simulink model "DC_MCC"  (R2018b)
settings: Solver=FixedStepDiscrete  StartTime=0.0  StopTime=11  RelTol=1e-3  EnableMultiTasking=on
PreLoadFcn:
  | assignin('base','Ts',5e-6)
InitFcn:
  | assignin('base','Ts',5e-6)
values from neighbouring files (symbols this model uses):
  Cn = 104    [MCC.m]
  f = (phi_0*In-Cn)/Omega_n    (= 0.0113704691797)    [MCC.m]
  J = 0.12    [MCC.m]
  kc = 0    [MCC.m]
  Ki = 15    [MCC.m]
  Kw = 8    [MCC.m]
  L = 6.3e-3    (= 0.0063)    [MCC.m]
  Laf = phi_0/Ifn    (= 0.693402070952)    [MCC.m]
  Lf = 0.75*Rf    (= 102.964285714)    [MCC.m]
  Nn = 3390    [MCC.m]
  Pn = 41.4e3    (= 41400)    [MCC.m]
  R = 0.64    [MCC.m]
  Rf = Uf/Ifn    (= 137.285714286)    [MCC.m]
  to_i = L/R    (= 0.00984375)    [MCC.m]
  to_w = J/f    (= 10.5536542163)    [MCC.m]
  Uf = 310    [MCC.m]
  Un = 600    [MCC.m]
undefined symbols (not defined in the file or in its folder): DiscIntNeverNeededParam, find_system, Ts
libraries: powerlib x22, powerlib_meascontrol x3, simulink_extras x1, simulink x1
(part 1 of 2)
Description:
  | Copyright 2008-2018 The MathWorks, Inc.
settings Model: ExtModeAutoUpdateStatusClock=off  Creator=MathWorks  LastModifiedBy=Louis
settings DataIOCC: InitialState=xFinal  SaveFormat=StructureWithTime  SignalLoggingSaveFormat=ModelDataLogs  SaveOutput=off  SignalLogging=off  SaveTime=off  SignalLoggingName=sigsOut
settings OptimizationCC: BooleanDataType=off  ExpressionDepthLimit=2147483647  InitFltsAndDblsToZero=on  EfficientMapNaN2IntZero=off  LifeSpan=inf  BufferReusableBoundary=off
settings DebuggingCC: UnderspecifiedInitializationDetection=Classic  MergeDetectMultiDrivingBlocksExec=none  CheckExecutionContextPreStartOutputMsg=on  CheckExecutionContextRuntimeOutputMsg=on  SignalResolutionControl=TryResolveAllWithWarning  MultiTaskDSMMsg=warning  MultiTaskCondExecSysMsg=none  FcnCallInpInsideContextMsg=warning  BusObjectLabelMismatch=none  AllowSymbolicDim=off  StateNameClashWarn=warning  SFUnexpectedBacktrackingDiag=warning  SFNoUnconditionalDefaultTransitionDiag=warning  SFExecutionAtInitializationDiag=none
settings HardwareCC: ProdBitPerPointer=32  ProdBitPerSizeT=32  ProdBitPerPtrDiffT=32  ProdLargestAtomicFloat=None  ProdIntDivRoundTo=Undefined  ProdEndianess=Unspecified  ProdWordSize=32  ProdHWDeviceType=32-bit Generic  TargetUnknown=on
settings ModelReferenceCC: PropagateSignalLabelsOutOfModel=off
settings SFSimCC: SimUseLocalCustomCode=off
settings RTWCC: RTWUseLocalCustomCode=off
settings CodeAppCC: StateflowObjectComments=on
settings GRTTargetCC: TargetLangStandard=C89/C90 (ANSI)  GeneratePreprocessorConditionals=Disable all  CombineOutputUpdateFcns=off  GRTInterface=on
settings ConfigComp: CovMetricSettings=dw  CovHtmlReporting=on  CovSaveCumulativeToWorkspaceVar=on  CovSaveSingleToWorkspaceVar=on  CovExternalEMLEnable=off  CovSFcnEnable=off
settings SimscapeCC: SimscapeNormalizeSystem=off

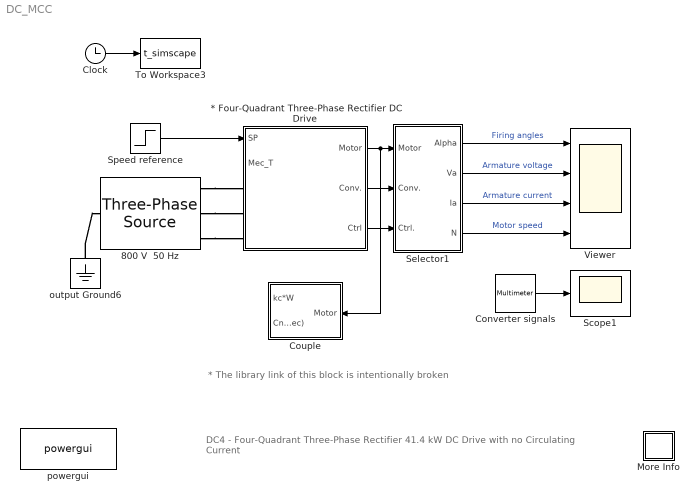
== system DC_MCC ==
  note: DC4 - Four-Quadrant Three-Phase Rectifier 41.4 kW DC Drive
      | with no Circulating Current
  note: * The library link of this block is intentionally broken
  * Four-Quadrant Three-Phase Rectifier DC Drive : Subsystem  mask(DC4){}
      mask init:
      | [X1,X1m,X2,X2m,X3,X4,Y1,Y1m,Y2,Y2m,Y3,Y4,color1,color2]=spsdrivelogo;
      mask Display:
      | patch([X1 X1m],[Y1 Y1m],color1);
      | patch(X3,Y3,color2);
      | plot([X1 X1m X2 X2m X3 X4],[Y1 Y1m Y2 Y2m Y3 Y4]);
      | text(0.5,0.3,'DC4*','HorizontalAlignment','center')
  800 V  50 Hz : powerlib/Electrical Sources/Three-Phase Source  InternalConnection=Yn  VoltagePhases=off  Voltage=800  PhaseAngle=0  Voltage_phases=[25e3 25e3 25e3]/sqrt(3)  PhaseAngles_phases=[0 -120 +120]  Frequency=50  NonIdealSource=on  SpecifyImpedance=off  Resistance=0.01  Inductance=0.1e-3  ShortCircuitLevel=0  BaseVoltage=0  XRratio=0  BusType=swing  Pref=0  Qref=0  Prefabc=0  Qrefabc=0  Qmin=-inf  Qmax=inf
      settings: SourceProductName=Simscape Electrical
  Clock : Clock
  Converter signals : powerlib/Measurements/Multimeter  PhasorSimulation=off  OutputType=Complex  sel=[10 20]  L=32  Gain=[1 1]  yselected={'Udc: * Four-Quadrant Three-Phase Rectifier DC Drive/Thyristor converter 1','Udc: * Four-Quadrant Three-Phase Rectifier DC Drive/Thyristor converter 2'};  PSBOutputType=1  PSBequivalent=0  AxesSetting=[0,0.1,-100,100]  Display=0  SavedBlockNames=-11
      settings: SourceProductName=Simscape Electrical
  Couple : Subsystem
  More Info : Subsystem
      settings: OpenFcn=showdemo(bdroot(gcb))
      mask Display: disp('?')
  Scope1 : Scope
  Selector1 : Subsystem
  Speed reference : Step  Time=4  After=Nn  SampleTime=0
  To Workspace3 : ToWorkspace  VariableName=t_simscape  SampleTime=-1
  Viewer : Scope  NumInputPorts=4
  output Ground6 : powerlib/Elements/Ground  LConnTagsString=a
      settings: SourceProductName=Simscape Electrical
  powergui : powerlib/powergui  Priority=2  SimulationMode=Discrete  SampleTime=Ts  frequency=60  Iterations=50  frequencyindice=50  Pbase=100e6  ErrMax=1e-4  UnitsV=kV  UnitsW=MW  buscounter=0  FunctionMessages=off  echomessages=off  EnableUseOfTLC=off  CurrentSourceSwitches=off  DisableSnubberDevices=off  DisableRonSwitches=off  DisableVfSwitches=off  DisplayEquations=off  SolverType=Tustin/Backward Euler (TBE)  Interpol=off  ExternalGateDelay=off  methode=off  Ts=0  x0status=blocks  SPID=off  SwTol=0  HookPort=off  RestoreLinks=warning  ResistiveCurrentMeasurement=off  Frange=[0:2:500]  Ylog=off  Xlog=on  ShowGrid=off  save=off  variable=ZData  structure=0  ZoomFFT=on  StartTime=0.0  cycles=1  DisplayStyle=1  fundamental=60  FreqAxis=off  MaxFrequency=1000  frequencyindicesteady=1  RmsSteady=1  display=off
  wires:
  Selector1/1(Alpha) -> Viewer/1  "Firing angles"
  Selector1/2(Va) -> Viewer/2  "Armature voltage"
  Selector1/3(Ia) -> Viewer/3  "Armature current"
  Selector1/4(N) -> Viewer/4  "Motor speed"
  * Four-Quadrant Three-Phase Rectifier DC Drive/1("Motor ") -> Couple/1(Motor), Selector1/1(Motor)
  * Four-Quadrant Three-Phase Rectifier DC Drive/2(Conv.) -> Selector1/2(Conv.)
  * Four-Quadrant Three-Phase Rectifier DC Drive/3(Ctrl) -> Selector1/3(Ctrl.)
  Speed reference/1 -> * Four-Quadrant Three-Phase Rectifier DC Drive/1(SP)
  Converter signals/1 -> Scope1/1
  Clock/1 -> To Workspace3/1
  connections:
  output Ground6/LConn1 -- 800 V  50 Hz/LConn1
  800 V  50 Hz/RConn1 -- * Four-Quadrant Three-Phase Rectifier DC Drive/LConn1
  800 V  50 Hz/RConn2 -- * Four-Quadrant Three-Phase Rectifier DC Drive/LConn2
  800 V  50 Hz/RConn3 -- * Four-Quadrant Three-Phase Rectifier DC Drive/LConn3

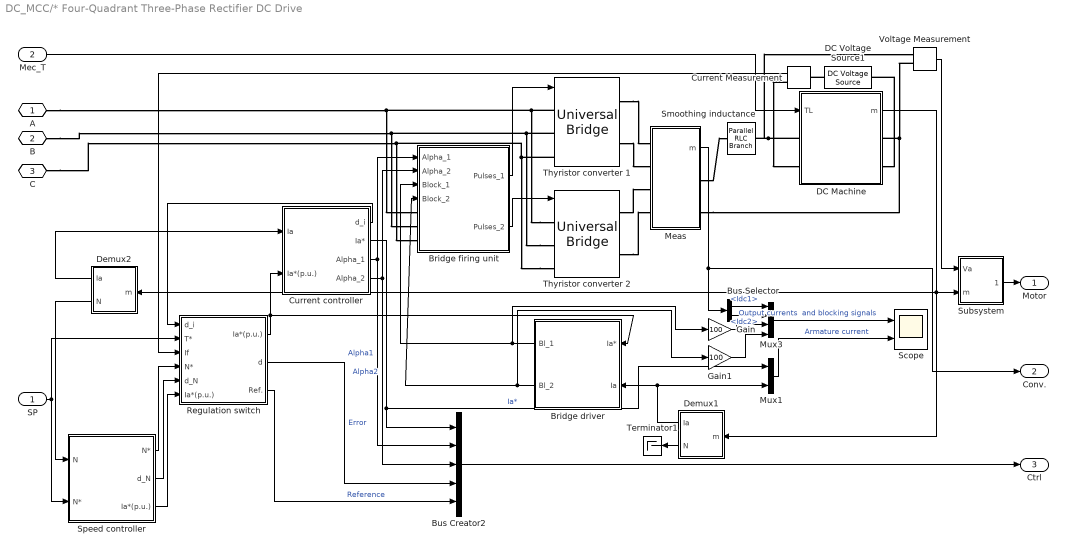
== system DC_MCC/* Four-Quadrant Three-Phase Rectifier DC Drive ==
  SP : Inport
  Mec_T : Inport  Port=2
  Bridge driver : Subsystem  mask(Bridge driver){P=Pn, V=Un, hyst=[-0.004 0.004], iazone=[0.003 0.003], irefzone=[-0.004 0.004], time=8e-3, sampling=100e-6}
      mask prompts: P "Base power (VA)"; V "Base voltage (V)"; hyst "Reference current hysteresis band [off on](p.u.)"; iazone "Armature current dead zone [low high] (p.u.)"; irefzone "Reference current dead zone [low high] (p.u.)"; time "Crossover timer delay (s)"; sampling "Controller sampling time (s)"
      mask help: This unit manages the bridge crossover process.
      mask init:
      | [X1,X1m,X2,X2m,X3,X4,Y1,Y1m,Y2,Y2m,Y3,Y4,color1,color2]=spsdrivelogo;
      | ib=P/V;
      mask Display:
      | patch([X1 X1m],[Y1 Y1m],color1);
      | patch(X3,Y3,color2);
      | plot([X1 X1m X2 X2m X3 X4],[Y1 Y1m Y2 Y2m Y3 Y4]);
  "Bridge firing unit " : Subsystem  mask(Bridge firing unit){x4=50, x9=20, Ts=Ts}
      mask prompts: x4 "Frequency of synchronisation voltages (Hz)"; x9 "Pulse width (deg.)"; Ts "Simulation time step (s)"
  Bus Creator2 : BusCreator  Inputs=5
  Bus Selector : BusSelector  OutputSignals=Idc1,Idc2
  Current Measurement : powerlib/Measurements/Current Measurement  Tag=PoWeRsYsTeMmEaSuReMeNt  PhasorSimulation=off  OutputType=Magnitude  PSBequivalent=0
      settings: SourceProductName=Simscape Electrical
  Current controller : Subsystem  Description=Current controller  mask(Current controller){Pb=Pn, Vb=Un, Kp=Ki, Ki=Ki/to_i, fci=100, lim=[20,160], sampling=100e-6, Ts=Ts}
      mask prompts: Pb "Base power (VA)"; Vb "Base voltage (V)"; Kp "Proportional gain"; Ki "Integral gain"; fci "Low-pass filter-Cut-off frequency (Hz)"; lim "Firing angle limits [ alpha_min alpha_max ] (deg.)"; sampling "Controller sampling time (s)"; Ts "Simulation time step (s)"
      mask help: This bloc implements a PI current regulator.
      mask init:
      | ib=Pb/Vb; lowlim=lim(1); highlim=lim(2);
      | [X1,X1m,X2,X2m,X3,X4,Y1,Y1m,Y2,Y2m,Y3,Y4,color1,color2]=spsdrivelogo;
      mask Display:
      | patch([X1 X1m],[Y1 Y1m],color1);
      | patch(X3,Y3,color2);
      | plot([X1 X1m X2 X2m X3 X4],[Y1 Y1m Y2 Y2m Y3 Y4]);
  DC Machine : Subsystem  LoadFcn=find_system(gcs,'FollowLinks', 'on', 'LookUnderMasks', 'all');  mask(Discrete DC machine){PresetModel=No, ShowDetailedParameters=on, RLa=[R L], RLf=[Rf Lf], Laf=Laf, J=J, Bm=f, Tf=0, w0=0, SampleTime=Ts}
      mask prompts: PresetModel "Preset  model"; ShowDetailedParameters "-----------------  Show detailed parameters -----------------"; RLa "Armature resistance and inductance [Ra (ohms) La (H) ]"; RLf "Field resistance and inductance [Rf (ohms) Lf (H) ]"; Laf "Field-armature mutual inductance Laf (H) :"; J "Total inertia J (kg.m^2)"; Bm "Viscous friction coefficient Bm (N.m.s)"; Tf "Coulomb friction torque Tf (N.m)"; w0 "Initial speed (rad/s) :"; SampleTime "Sample Time"
      mask help: This block implements a separately excited DC machine. Access is provided to the field connections so that the machine can be used as a shunt-connected or a series-connected DC machine.
      mask init:
      | Ra=RLa(1); La=RLa(2);
      | 
      | Rf=RLf(1); Lf=RLf(2);
      settings: AttributesFormatString=\n
      mask Help: helpview(psbhelp)
      mask TypeOptions PresetModel: No | 01: 5Hp 240Vdc 1750RPM Field:300Vdc | 02: 5Hp 500Vdc 1750RPM Field:300Vdc | 03: 10Hp 240Vdc 1750RPM Field:300Vdc | 04: 10Hp 500Vdc 1750RPM Field:300Vdc | 05: 20Hp 240Vdc 1750RPM Field:300Vdc | 06: 20Hp 500Vdc 1750RPM Field:300Vdc | 07: 30Hp 240Vdc 1750RPM Field:300Vdc | 08: 30Hp 500Vdc 1750RPM Field:300Vdc | 09: 40Hp 240Vdc 1750RPM Field:300Vdc | 10: 40Hp 500Vdc 1750RPM Field:300Vdc | 11: 50Hp 240Vdc 1750RPM Field:300Vdc | 12: 50Hp 500Vdc 1750RPM Field:300Vdc | 13: 75Hp 500Vdc 1750RPM Field:300Vdc | 14: 100Hp 500Vdc 1750RPM Field:300Vdc | 15: 125Hp 500Vdc 1750RPM Field:300Vdc | 16: 150Hp 500Vdc 1750RPM Field:300Vdc | 17: 175Hp 500Vdc 1750RPM Field:300Vdc | 18: 200Hp 500Vdc 1750RPM Field:300Vdc | 19: 225Hp 500Vdc 1750RPM Field:300Vdc | 20: 250Hp 500Vdc 1750RPM Field:300Vdc
      mask Callback PresetModel: powericon('DCMachineCback',gcb,'Discrete');
      mask Callback ShowDetailedParameters: powericon('DCMachineCback',gcb,'Discrete');
      mask Display:
      | plot(-80,-80,80,80,[0,9,18,24,29,30,29,24,18,9,0,-9,-18,-24,-29,-30,-29,-24,-18,-9,0],[30,29,24,18,9,0,-9,-18,-24,-29,-30,-29,-24,-18,-9,0,9,18,24,29,30],[-29,-35,-35,-29],[-8,-8,8,8],[29,35,35,29],[-8,-8,8,8],[-35,-55],[0,0],[35,55],[0,0],[-78,-50,-50,-49,-45,-39,-33,-26,-21,-18,-17,-19,-22,-22,-26,-27,-25,-22,-16,-9,-3,2,6,6,4,1,1,-3,-4,-2,2,7,14,20,26,29,30,28,24,24,21,20,21,25,31,37,44,49,50,50,50,78]*.7,[58,58,57.2,49.2,42.8,38.8,38,39.6,44.4,51.6,59.6,67.6,72.4,72.4,65.2,57.2,49.2,42.8,38.8,38,39.6,44.4,51.6,59.6,67.6,72.4,72.4,65.2,57.2,49.2,42.8,38.8,38,39.6,44.4,51.6,59.6,67.6,72.4,72.4,65.2,57.2,49.2,42.8,38.8,38,39.6,44.4,51.6,58,58,58]*.6-85 );
      | 
      | disp('dc')
      | 
      | color('blue');
      | 
      | plot([-50,-10,-10],[50,50,30]);
      | 
      | plot([50,10,10],[50,50,30]);
  DC Voltage Source1 : powerlib/Electrical Sources/DC Voltage Source  Description=source block  Amplitude=Uf  Measurements=None
      settings: AttributesFormatString=\n  SourceProductName=Simscape Electrical
  Demux1 : Subsystem
  Demux2 : Subsystem
  Gain : Gain  Gain=100  SaturateOnIntegerOverflow=on  OutDataTypeStr=Inherit: Same as input  ParamDataTypeStr=Inherit: Same as input
  Gain1 : Gain  Gain=100  SaturateOnIntegerOverflow=on  OutDataTypeStr=Inherit: Same as input  ParamDataTypeStr=Inherit: Same as input
  Meas : Subsystem
  Mux1 : Mux  Inputs=2
  Mux3 : Mux
  Regulation switch : Subsystem  mask(Regulation switch){Swk=Speed regulation, P=Pn, V=Un, Laf=Laf, lim=1, sampling=100e-6, Ts=Ts}
      mask prompts: Swk "Regulation mode"; P "Base power (VA)"; V "Base voltage (V)"; Laf "Field-armature mutual inductance Laf (H)"; lim "Current ref. limit (p.u.)"; sampling "Controller sampling time (s)"; Ts "Simulation time step (s)"
      mask help: This block allows the user to choose between speed or torque regulation.
      mask init:
      | ib=P/V;
      | [X1,X1m,X2,X2m,X3,X4,Y1,Y1m,Y2,Y2m,Y3,Y4,color1,color2]=spsdrivelogo;
      mask TypeOptions Swk: Speed regulation | Torque regulation
      mask Display:
      | patch([X1 X1m],[Y1 Y1m],color1);
      | patch(X3,Y3,color2);
      | plot([X1 X1m X2 X2m X3 X4],[Y1 Y1m Y2 Y2m Y3 Y4]);
  Scope : Scope  NumInputPorts=2
  Smoothing inductance : powerlib/Elements/Parallel RLC Branch  LConnTagsString=a  RConnTagsString=__new0  BranchType=L  Resistance=1.0  Inductance=10e-3  SetiL0=off  InitialCurrent=0  Capacitance=1.0  Setx0=off  InitialVoltage=0  Measurements=None
      settings: SourceProductName=Simscape Electrical
  Speed controller : Subsystem  mask(Speed controller){wb=Nn, ramp=[-Nn,Nn], Is=0, Kp=Kw, Ki=Kw/to_w, lim=1, fcw=40, sampling=100e-6, Ts=Ts}
      mask prompts: wb "Base speed (rpm)"; ramp "Speed reference ramp (rpm/s) [deceleration,acceleration]"; Is "Initial speed reference (rpm)"; Kp "Proportional gain"; Ki "Integral gain"; lim "Current ref. limit (p.u.)"; fcw "Low-pass filter-Cut-off frequency (Hz)"; sampling "Controller sampling time (s)"; Ts "Simulation time step (s)"
      mask help: This bloc implements a PI speed regulator.
      mask init:
      | [X1,X1m,X2,X2m,X3,X4,Y1,Y1m,Y2,Y2m,Y3,Y4,color1,color2]=spsdrivelogo;
      mask Display:
      | patch([X1 X1m],[Y1 Y1m],color1);
      | patch(X3,Y3,color2);
      | plot([X1 X1m X2 X2m X3 X4],[Y1 Y1m Y2 Y2m Y3 Y4]);
  Subsystem : Subsystem
  Terminator1 : Terminator
  Thyristor converter 1 : powerlib/Power Electronics/Universal Bridge  Arms=3  SnubberResistance=9e3  SnubberCapacitance=900e-9  Device=Thyristors  Ron=1e-3  Lon=0  ForwardVoltages="[  0,  0  ]"  ForwardVoltage=1.3  GTOparameters=[ 10e-6, 20e-6 ]  IGBTparameters=[ 1e-6 , 2e-6 ]  Measurements=All voltages and currents  Measurements_2=None  converterType=Rectifier
      settings: SourceProductName=Simscape Electrical
  Thyristor converter 2 : powerlib/Power Electronics/Universal Bridge  Arms=3  SnubberResistance=9e3  SnubberCapacitance=900e-9  Device=Thyristors  Ron=1e-3  Lon=0  ForwardVoltages="[  0,  0  ]"  ForwardVoltage=1.3  GTOparameters=[ 10e-6, 20e-6 ]  IGBTparameters=[ 1e-6 , 2e-6 ]  Measurements=All voltages and currents  Measurements_2=None  converterType=Inverter
      settings: SourceProductName=Simscape Electrical
  Voltage Measurement : powerlib/Measurements/Voltage Measurement  Tag=PoWeRsYsTeMmEaSuReMeNt  PhasorSimulation=off  OutputType=Magnitude  PSBequivalent=0
      settings: SourceProductName=Simscape Electrical
  A : PMIOPort  Side=Left
  B : PMIOPort  Port=2  Side=Left
  C : PMIOPort  Port=3  Side=Left
  "Motor " : Outport
  Conv. : Outport  Port=2
  Ctrl : Outport  Port=3
  wires:
  Current controller/4(Alpha_2) -> "Bridge firing unit "/2(Alpha_2), Bus Creator2/3  "Alpha2"
  Current controller/3(Alpha_1) -> "Bridge firing unit "/1(Alpha_1), Bus Creator2/2  "Alpha1"
  Regulation switch/3(Ref.) -> Bus Creator2/5  "Reference"
  Current controller/1(d_i) -> Regulation switch/1(d_i)
  Current controller/2(Ia*) -> Mux1/1, Bus Creator2/1  "Ia*"
  Speed controller/1(" N*") -> Regulation switch/4(N*)
  Speed controller/2(d_N) -> Regulation switch/5(d_N)
  Speed controller/3(Ia*(p.u.)) -> Regulation switch/6(Ia*(p.u.))
  Regulation switch/1(" Ia*(p.u.)") -> Current controller/2(Ia*(p.u.)), Bridge driver/1(Ia*)
  Bus Creator2/1 -> Ctrl/1
  Subsystem/1(Motor) -> "Motor "/1
  SP/1 -> Regulation switch/2(T*), Speed controller/2(N*)
  Demux2/1(Ia) -> Current controller/1(Ia)
  Demux2/2(N) -> Speed controller/1(N)
  Current Measurement/1 -> Regulation switch/3(If)
  Mec_T/1 -> DC Machine/1(TL)
  Voltage Measurement/1 -> Subsystem/1(Va)
  DC Machine/1(m) -> Demux1/1(m), Demux2/1(m), Subsystem/2(m)
  "Bridge firing unit "/1(Pulses_1) -> Thyristor converter 1/1
  "Bridge firing unit "/2(Pulses_2) -> Thyristor converter 2/1
  Demux1/1(Ia) -> Bridge driver/2(Ia), Mux1/2
  Demux1/2(N) -> Terminator1/1
  Bridge driver/1(Bl_1) -> "Bridge firing unit "/3(Block_1), Gain/1
  Bridge driver/2(Bl_2) -> "Bridge firing unit "/4(Block_2), Gain1/1
  Mux3/1 -> Scope/1  "Output currents  and blocking signals"
  Mux1/1 -> Scope/2  "Armature current"
  Gain1/1 -> Mux3/4
  Gain/1 -> Mux3/3
  Meas/1("m ") -> Conv./1, Bus Selector/1
  Bus Selector/1 -> Mux3/1  "<Idc1>"
  Bus Selector/2 -> Mux3/2  "<Idc2>"
  Regulation switch/2(d) -> Bus Creator2/4  "Error"
  connections:
  DC Machine/RConn2 -- DC Voltage Source1/LConn1
  DC Voltage Source1/RConn1 -- Current Measurement/LConn1
  Thyristor converter 2/LConn1 -- Thyristor converter 1/LConn1 -- "Bridge firing unit "/LConn1 -- A/RConn1
  Thyristor converter 2/LConn2 -- Thyristor converter 1/LConn2 -- "Bridge firing unit "/LConn2 -- B/RConn1
  Thyristor converter 2/LConn3 -- Thyristor converter 1/LConn3 -- "Bridge firing unit "/LConn3 -- C/RConn1
  Current Measurement/RConn1 -- DC Machine/LConn2
  Voltage Measurement/LConn2 -- DC Machine/RConn1 -- Meas/RConn2
  DC Machine/LConn1 -- Voltage Measurement/LConn1 -- Smoothing inductance/RConn1
  Meas/RConn1 -- Smoothing inductance/LConn1
  Thyristor converter 1/RConn1 -- Meas/LConn1
  Thyristor converter 1/RConn2 -- Meas/LConn2
  Thyristor converter 2/RConn1 -- Meas/LConn3
  Thyristor converter 2/RConn2 -- Meas/LConn4

== system DC_MCC/Couple ==
  Motor : Inport
  Demux : Demux  Outputs=5
  Gain1 : Gain  Gain=2*pi/60
  Gain2 : Gain  Gain=kc
  Step : Step  Time=6  After=Cn  SampleTime=0
  kc*W : Outport
  Cn (6sec) : Outport  Port=2
  wires:
  Motor/1 -> Demux/1
  Demux/2 -> Gain1/1
  Gain1/1 -> Gain2/1
  Gain2/1 -> kc*W/1
  Step/1 -> Cn (6sec)/1

== system DC_MCC/More Info ==

== system DC_MCC/Selector1 ==
  Motor : Inport
  Conv. : Inport  Port=2
  Ctrl. : Inport  Port=3
  Bus Selector1 : BusSelector  OutputSignals=Ia*,Reference,Alpha1,Alpha2
  Bus Selector3 : BusSelector  OutputSignals=Armature Voltage (V),Armature current ia (A),Speed (rpm)
  Mux1 : Mux  Inputs=2
  Mux2 : Mux  Inputs=2
  Mux4 : Mux  Inputs=2
  Terminator : Terminator
  Alpha : Outport
  Va : Outport  Port=2
  Ia : Outport  Port=3
  N : Outport  Port=4
  wires:
  Mux2/1 -> Ia/1
  Mux4/1 -> N/1
  Mux1/1 -> Alpha/1
  Motor/1 -> Bus Selector3/1
  Bus Selector3/1 -> Va/1  "<Armature Voltage (V)>"
  Ctrl./1 -> Bus Selector1/1
  Bus Selector1/1 -> Mux2/2  "<Ia*>"
  Bus Selector1/2 -> Mux4/2  "<Reference>"
  Bus Selector1/3 -> Mux1/1  "<Alpha1>"
  Bus Selector1/4 -> Mux1/2  "<Alpha2>"
  Bus Selector3/2 -> Mux2/1  "<Armature current ia (A)>"
  Bus Selector3/3 -> Mux4/1  "<Speed (rpm)>"
  Conv./1 -> Terminator/1

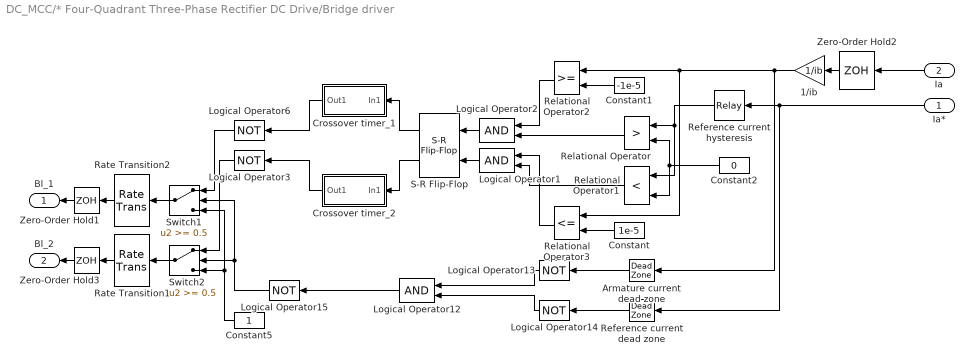
== system DC_MCC/* Four-Quadrant Three-Phase Rectifier DC Drive/Bridge driver ==
  Ia* : Inport
  Ia : Inport  Port=2
  1/ib : Gain  Gain=1/ib  SaturateOnIntegerOverflow=on  OutDataTypeStr=Inherit: Same as input  ParamDataTypeStr=Inherit: Same as input
  Armature current dead zone : DeadZone  LowerValue=iazone(1)  UpperValue=iazone(2)  SaturateOnIntegerOverflow=on
  Constant : Constant  Value=1e-5
  Constant1 : Constant  Value=-1e-5
  Constant2 : Constant  Value=0
  Constant5 : Constant
  Crossover timer_1 : Subsystem
  Crossover timer_2 : Subsystem
  Logical Operator1 : Logic
  Logical Operator12 : Logic
  Logical Operator{3,6,13..15} (5 alike) : Logic  Operator=NOT
  Logical Operator2 : Logic
  Rate Transition1 : RateTransition
  Rate Transition2 : RateTransition
  Reference current hysteresis : Relay  OnSwitchValue=hyst(2)  OffSwitchValue=hyst(1)  OffOutputValue=-1
  Reference current dead zone : DeadZone  LowerValue=irefzone(1)  UpperValue=irefzone(2)  SaturateOnIntegerOverflow=on
  Relational Operator : RelationalOperator  Operator=>  RndMeth=Nearest  InputSameDT=on
  Relational Operator1 : RelationalOperator  Operator=<  RndMeth=Nearest  InputSameDT=on
  Relational Operator2 : RelationalOperator  RndMeth=Nearest  InputSameDT=on
  Relational Operator3 : RelationalOperator  Operator=<=  RndMeth=Nearest  InputSameDT=on
  S-R Flip-Flop : simulink_extras/Flip Flops/S-R Flip-Flop  initial_condition=0
  Switch1 : Switch  Threshold=0.5  SaturateOnIntegerOverflow=on  InputSameDT=on
  Switch2 : Switch  Threshold=0.5  SaturateOnIntegerOverflow=on  InputSameDT=on
  Zero-Order Hold1 : ZeroOrderHold  SampleTime=Ts
  Zero-Order Hold2 : ZeroOrderHold  SampleTime=sampling
  Zero-Order Hold3 : ZeroOrderHold  SampleTime=Ts
  Bl_1 : Outport
  Bl_2 : Outport  Port=2
  wires:
  Relational Operator/1 -> Logical Operator2/2
  Relational Operator1/1 -> Logical Operator1/2
  Relational Operator3/1 -> Logical Operator1/1
  Relational Operator2/1 -> Logical Operator2/1
  Logical Operator6/1 -> Switch1/1
  Logical Operator3/1 -> Switch2/1
  Constant5/1 -> Switch2/3, Switch1/3
  Armature current dead zone/1 -> Logical Operator13/1
  Reference current dead zone/1 -> Logical Operator14/1
  Logical Operator13/1 -> Logical Operator12/1
  Logical Operator14/1 -> Logical Operator12/2
  Logical Operator15/1 -> Switch2/2, Switch1/2
  Logical Operator1/1 -> S-R Flip-Flop/2
  Ia*/1 -> Reference current hysteresis/1, Reference current dead zone/1
  Logical Operator12/1 -> Logical Operator15/1
  Constant1/1 -> Relational Operator2/2
  Constant/1 -> Relational Operator3/2
  Constant2/1 -> Relational Operator1/2, Relational Operator/2
  Ia/1 -> Zero-Order Hold2/1
  Logical Operator2/1 -> S-R Flip-Flop/1
  S-R Flip-Flop/2 -> Crossover timer_2/1(In1)
  S-R Flip-Flop/1 -> Crossover timer_1/1(In1)
  Zero-Order Hold1/1 -> Bl_1/1
  Crossover timer_2/1(Out1) -> Logical Operator3/1
  Zero-Order Hold3/1 -> Bl_2/1
  Switch2/1 -> Rate Transition1/1
  Rate Transition1/1 -> Zero-Order Hold3/1
  Crossover timer_1/1(Out1) -> Logical Operator6/1
  Zero-Order Hold2/1 -> 1/ib/1
  1/ib/1 -> Relational Operator3/1, Relational Operator2/1, Armature current dead zone/1
  Switch1/1 -> Rate Transition2/1
  Rate Transition2/1 -> Zero-Order Hold1/1
  Reference current hysteresis/1 -> Relational Operator/1, Relational Operator1/1

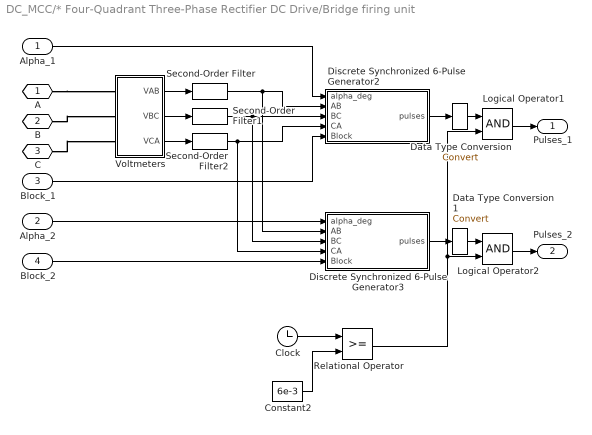
== system DC_MCC/* Four-Quadrant Three-Phase Rectifier DC Drive/Bridge firing unit  ==
  Alpha_1 : Inport
  Alpha_2 : Inport  Port=2
  Block_1 : Inport  Port=3
  Block_2 : Inport  Port=4
  Clock : Clock
  Constant2 : Constant  Value=6e-3
  Data Type Conversion : DataTypeConversion  SaturateOnIntegerOverflow=on  RndMeth=Zero
  Data Type Conversion1 : DataTypeConversion  SaturateOnIntegerOverflow=on  RndMeth=Zero
  Discrete Synchronized 6-Pulse Generator2 : Subsystem  mask(Discrete Synchronized 6-pulse generator){freq=x4, pwidth=x9, Double_Pulse=on, Ts=Ts}
      mask prompts: freq "Frequency of sync. voltages (Hz):"; pwidth "Pulse width (degrees) :"; Double_Pulse "Double pulsing"; Ts "Time step (s) :"
      mask help:
      | Use this block to fire the 6 thyristors of a 6-pulse converter.
      |
      | The output is a vector of 6 pulses (0-1) individually synchronized on the 6 commutation voltages. Pulses are generated alpha degrees after the increasing zero-crossings of the commutation voltages.
      |
      | Input 1 is  the alpha firing signal (degrees).
      | Inputs 2, 3 and 4 are the synchronization voltages AB BC CA which should be in phase with the 3 phase-phase voltages at the converter terminals.
      | Input 5: Frequency of the synchronization voltages (use a constant or the Freq PLL output)
      | Input 6 allows  blocking of the pulses when the applied signal is non zero.
      |
      | When the 'Douple pulsing' option is checked, two pulses are sent to each thyristor: a 1st pulse when the aplha angle is reached, then a 2nd pulse 60 degrees later, when the next thyristor is fired.
      mask Display: plot(0,0,100,100,[80 62 62 47 47 30],[40 40 60 60 40 40]-5)
  Discrete Synchronized 6-Pulse Generator3 : Subsystem  mask(Discrete Synchronized 6-pulse generator){freq=x4, pwidth=x9, Double_Pulse=on, Ts=Ts}
      mask prompts: freq "Frequency of sync. voltages (Hz):"; pwidth "Pulse width (degrees) :"; Double_Pulse "Double pulsing"; Ts "Time step (s) :"
      mask help:
      | Use this block to fire the 6 thyristors of a 6-pulse converter.
      |
      | The output is a vector of 6 pulses (0-1) individually synchronized on the 6 commutation voltages. Pulses are generated alpha degrees after the increasing zero-crossings of the commutation voltages.
      |
      | Input 1 is  the alpha firing signal (degrees).
      | Inputs 2, 3 and 4 are the synchronization voltages AB BC CA which should be in phase with the 3 phase-phase voltages at the converter terminals.
      | Input 5: Frequency of the synchronization voltages (use a constant or the Freq PLL output)
      | Input 6 allows  blocking of the pulses when the applied signal is non zero.
      |
      | When the 'Douple pulsing' option is checked, two pulses are sent to each thyristor: a 1st pulse when the aplha angle is reached, then a 2nd pulse 60 degrees later, when the next thyristor is fired.
      mask Display: plot(0,0,100,100,[80 62 62 47 47 30],[40 40 60 60 40 40]-5)
  Logical Operator1 : Logic
  Logical Operator2 : Logic
  Relational Operator : RelationalOperator  RndMeth=Nearest  InputSameDT=on
  Second-Order Filter : powerlib_meascontrol/Filters/Second-Order Filter  FilterType=Bandpass  Fo=x4  Zeta=0.25  Ts=Ts  Initialize=off  Vac_Init="[0,  0,  60]"  Vdc_Init=0  PlotResponse=off  FreqRange=[0, 500, 1]
      settings: SourceProductName=Simscape Electrical  SourceProductBaseCode=PS
  Second-Order Filter1 : powerlib_meascontrol/Filters/Second-Order Filter  FilterType=Bandpass  Fo=x4  Zeta=0.25  Ts=Ts  Initialize=on  Vac_Init=[0.8 -25 60]  Vdc_Init=-0.4  PlotResponse=off  FreqRange=[0, 500, 1]
      settings: SourceProductName=Simscape Electrical  SourceProductBaseCode=PS
  Second-Order Filter2 : powerlib_meascontrol/Filters/Second-Order Filter  FilterType=Bandpass  Fo=x4  Zeta=0.25  Ts=Ts  Initialize=on  Vac_Init=[0.8 -25 60]  Vdc_Init=-0.4  PlotResponse=off  FreqRange=[0, 500, 1]
      settings: SourceProductName=Simscape Electrical  SourceProductBaseCode=PS
  Voltmeters : Subsystem
  A : PMIOPort  Side=Left
  B : PMIOPort  Port=2  Side=Left
  C : PMIOPort  Port=3  Side=Left
  Pulses_1 : Outport
  Pulses_2 : Outport  Port=2
  wires:
  Discrete Synchronized 6-Pulse Generator3/1(pulses) -> Data Type Conversion1/1
  Logical Operator2/1 -> Pulses_2/1
  Discrete Synchronized 6-Pulse Generator2/1(pulses) -> Data Type Conversion/1
  Logical Operator1/1 -> Pulses_1/1
  Relational Operator/1 -> Logical Operator1/2, Logical Operator2/2
  Constant2/1 -> Relational Operator/2
  Clock/1 -> Relational Operator/1
  Voltmeters/1(VAB) -> Second-Order Filter/1
  Voltmeters/2(VBC) -> Second-Order Filter1/1
  Voltmeters/3(VCA) -> Second-Order Filter2/1
  Alpha_1/1 -> Discrete Synchronized 6-Pulse Generator2/1(alpha_deg)
  Second-Order Filter/1 -> Discrete Synchronized 6-Pulse Generator2/2(AB), Discrete Synchronized 6-Pulse Generator3/2(AB)
  Second-Order Filter1/1 -> Discrete Synchronized 6-Pulse Generator2/3(BC), Discrete Synchronized 6-Pulse Generator3/3(BC)
  Second-Order Filter2/1 -> Discrete Synchronized 6-Pulse Generator2/4(CA), Discrete Synchronized 6-Pulse Generator3/4(CA)
  Alpha_2/1 -> Discrete Synchronized 6-Pulse Generator3/1(alpha_deg)
  Block_1/1 -> Discrete Synchronized 6-Pulse Generator2/5(Block)
  Block_2/1 -> Discrete Synchronized 6-Pulse Generator3/5(Block)
  Data Type Conversion/1 -> Logical Operator1/1
  Data Type Conversion1/1 -> Logical Operator2/1
  connections:
  A/RConn1 -- Voltmeters/LConn1
  B/RConn1 -- Voltmeters/LConn2
  C/RConn1 -- Voltmeters/LConn3

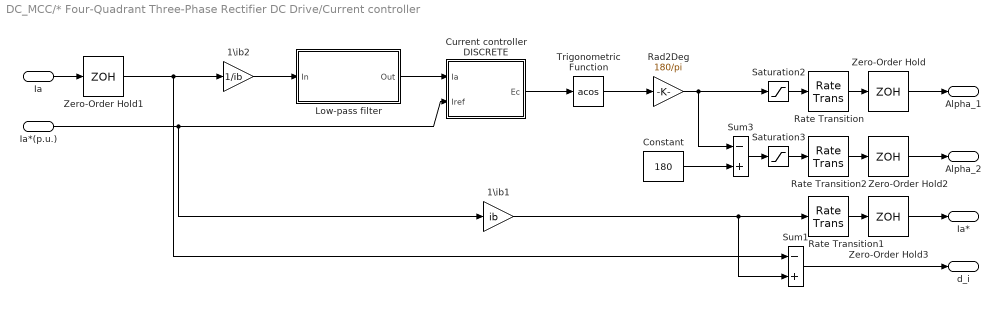
== system DC_MCC/* Four-Quadrant Three-Phase Rectifier DC Drive/Current controller ==
  Ia : Inport
  Ia*(p.u.) : Inport  Port=2
  1\ib1 : Gain  Gain=ib  SaturateOnIntegerOverflow=on  OutDataTypeStr=Inherit: Same as input  ParamDataTypeStr=Inherit: Same as input
  1\ib2 : Gain  Gain=1/ib  SaturateOnIntegerOverflow=on  OutDataTypeStr=Inherit: Same as input  ParamDataTypeStr=Inherit: Same as input
  Constant : Constant  Value=180
  Current controller DISCRETE : Subsystem  mask(PI controller){Kp=Kp, Ki=Ki, Ts=sampling}
      mask prompts: Kp "Proportional gain (Kp)"; Ki "Integral gain (Ki)"; Ts "Sample time (s) :"
      mask help: Proportional-Integral Speed Controller
      mask Display: plot(0,0,100,100,[35,35,65],[70,30,30],[35,65],[45,60])
  Low-pass filter : Subsystem
  Rad2Deg : Gain  Gain=180/pi  SaturateOnIntegerOverflow=on  OutDataTypeStr=Inherit: Same as input  ParamDataTypeStr=Inherit: Same as input
  Rate Transition : RateTransition
  Rate Transition1 : RateTransition
  Rate Transition2 : RateTransition
  Saturation2 : Saturate  UpperLimit=highlim  LowerLimit=lowlim
  Saturation3 : Saturate  UpperLimit=highlim  LowerLimit=lowlim
  Sum1 : Sum  Inputs=-+  SaturateOnIntegerOverflow=on  InputSameDT=on  OutDataTypeStr=Inherit: Same as first input
  Sum3 : Sum  Inputs=-+  SaturateOnIntegerOverflow=on  InputSameDT=on  OutDataTypeStr=Inherit: Same as first input
  Trigonometric Function : Trigonometry  Operator=acos
  Zero-Order Hold : ZeroOrderHold  SampleTime=Ts
  Zero-Order Hold1 : ZeroOrderHold  SampleTime=sampling
  Zero-Order Hold2 : ZeroOrderHold  SampleTime=Ts
  Zero-Order Hold3 : ZeroOrderHold  SampleTime=Ts
  d_i : Outport
  Ia* : Outport  Port=2
  Alpha_1 : Outport  Port=3
  Alpha_2 : Outport  Port=4
  wires:
  Rad2Deg/1 -> Saturation2/1, Sum3/1
  Trigonometric Function/1 -> Rad2Deg/1
  Current controller DISCRETE/1(Ec) -> Trigonometric Function/1
  Ia*(p.u.)/1 -> 1\ib1/1, Current controller DISCRETE/2(Iref)
  Low-pass filter/1(Out) -> Current controller DISCRETE/1(Ia)
  1\ib2/1 -> Low-pass filter/1(In)
  Zero-Order Hold1/1 -> Sum1/1, 1\ib2/1
  Ia/1 -> Zero-Order Hold1/1
  Sum1/1 -> d_i/1
  Zero-Order Hold/1 -> Alpha_1/1
  Saturation2/1 -> Rate Transition/1
  Rate Transition1/1 -> Zero-Order Hold3/1
  Zero-Order Hold3/1 -> Ia*/1
  Rate Transition/1 -> Zero-Order Hold/1
  1\ib1/1 -> Sum1/2, Rate Transition1/1
  Saturation3/1 -> Rate Transition2/1
  Zero-Order Hold2/1 -> Alpha_2/1
  Constant/1 -> Sum3/2
  Rate Transition2/1 -> Zero-Order Hold2/1
  Sum3/1 -> Saturation3/1

== system DC_MCC/* Four-Quadrant Three-Phase Rectifier DC Drive/DC Machine ==
  TL : Inport
  FCEM : powerlib/Electrical Sources/Controlled Voltage Source  Description=source block  Initialize=on  Source_Type=AC  Amplitude=0  Phase=0  Frequency=0  Measurements=None
      settings: SourceProductName=Simscape Electrical
  Measurement list : Subsystem
  Mechanics : Subsystem
  Ra La : powerlib/Elements/Series RLC Branch  LConnTagsString=__new0  RConnTagsString=__new0  BranchType=RL  Resistance=Ra  Inductance=La  SetiL0=off  InitialCurrent=0  Capacitance=1.0  Setx0=off  InitialVoltage=0  Measurements=None
      settings: SourceProductName=Simscape Electrical
  Rf  Lf : powerlib/Elements/Series RLC Branch  LConnTagsString=__new0  RConnTagsString=__new0  BranchType=RL  Resistance=Rf  Inductance=Lf  SetiL0=off  InitialCurrent=0  Capacitance=1.0  Setx0=off  InitialVoltage=0  Measurements=None
      settings: SourceProductName=Simscape Electrical
  iA : powerlib/Measurements/Current Measurement  PhasorSimulation=off  OutputType=Magnitude  PSBequivalent=0
      settings: SourceProductName=Simscape Electrical
  iF : powerlib/Measurements/Current Measurement  PhasorSimulation=off  OutputType=Magnitude  PSBequivalent=0
      settings: SourceProductName=Simscape Electrical
  A+ : PMIOPort  Side=Left
  A- : PMIOPort  Port=2  Side=Right
  F+ : PMIOPort  Port=3  Side=Left
  F- : PMIOPort  Port=4  Side=Right
  m : Outport
  wires:
  Measurement list/1(Out1) -> m/1
  Mechanics/1(m) -> Measurement list/1(In1)
  TL/1 -> Mechanics/1(TL)
  iF/1 -> Mechanics/3(iF)
  Mechanics/2(FCEM) -> FCEM/1
  iA/1 -> Mechanics/2(iA)
  connections:
  F-/RConn1 -- Rf  Lf/RConn1
  F+/RConn1 -- iF/LConn1
  A-/RConn1 -- FCEM/LConn1
  A+/RConn1 -- iA/LConn1
  iF/RConn1 -- Rf  Lf/LConn1
  iA/RConn1 -- Ra La/LConn1
  FCEM/RConn1 -- Ra La/RConn1

== system DC_MCC/* Four-Quadrant Three-Phase Rectifier DC Drive/Demux1 ==
  m : Inport
  Demux : Demux
  Rad2Rpm : Gain  Gain=30/pi  SaturateOnIntegerOverflow=on  OutDataTypeStr=Inherit: Same as input  ParamDataTypeStr=Inherit: Same as input
  Terminator : Terminator
  Terminator1 : Terminator
  Ia : Outport
  N : Outport  Port=2
  wires:
  Demux/4 -> Terminator1/1
  Demux/3 -> Terminator/1
  m/1 -> Demux/1
  Demux/2 -> Ia/1
  Demux/1 -> Rad2Rpm/1
  Rad2Rpm/1 -> N/1

== system DC_MCC/* Four-Quadrant Three-Phase Rectifier DC Drive/Demux2 ==
  m : Inport
  Demux : Demux
  Rad2Rpm : Gain  Gain=30/pi  SaturateOnIntegerOverflow=on  OutDataTypeStr=Inherit: Same as input  ParamDataTypeStr=Inherit: Same as input
  Terminator : Terminator
  Terminator1 : Terminator
  Ia : Outport
  N : Outport  Port=2
  wires:
  Demux/4 -> Terminator1/1
  Demux/3 -> Terminator/1
  m/1 -> Demux/1
  Demux/2 -> Ia/1
  Demux/1 -> Rad2Rpm/1
  Rad2Rpm/1 -> N/1

== system DC_MCC/* Four-Quadrant Three-Phase Rectifier DC Drive/Meas ==
  Bus Creator2 : BusCreator  Inputs=4
  Current Measurement3 : powerlib/Measurements/Current Measurement  Tag=PoWeRsYsTeMmEaSuReMeNt  PhasorSimulation=off  OutputType=Magnitude  PSBequivalent=0
      settings: SourceProductName=Simscape Electrical
  Current Measurement4 : powerlib/Measurements/Current Measurement  Tag=PoWeRsYsTeMmEaSuReMeNt  PhasorSimulation=off  OutputType=Magnitude  PSBequivalent=0
      settings: SourceProductName=Simscape Electrical
  Voltage Measurement1 : powerlib/Measurements/Voltage Measurement  Tag=PoWeRsYsTeMmEaSuReMeNt  PhasorSimulation=off  OutputType=Magnitude  PSBequivalent=0
      settings: SourceProductName=Simscape Electrical
  Voltage Measurement2 : powerlib/Measurements/Voltage Measurement  Tag=PoWeRsYsTeMmEaSuReMeNt  PhasorSimulation=off  OutputType=Magnitude  PSBequivalent=0
      settings: SourceProductName=Simscape Electrical
  1+ : PMIOPort  Side=Left
  1_out : PMIOPort  Port=2  Side=Right
  1- : PMIOPort  Port=3  Side=Left
  2+ : PMIOPort  Port=4  Side=Left
  2_out : PMIOPort  Port=5  Side=Right
  2- : PMIOPort  Port=6  Side=Left
  "m " : Outport
  wires:
  Voltage Measurement1/1 -> Bus Creator2/1  "Vdc1"
  Voltage Measurement2/1 -> Bus Creator2/2  "Vdc2"
  Current Measurement4/1 -> Bus Creator2/3  "Idc1"
  Current Measurement3/1 -> Bus Creator2/4  "Idc2"
  Bus Creator2/1 -> "m "/1
  connections:
  1+/RConn1 -- Current Measurement4/LConn1 -- Voltage Measurement1/LConn1
  2_out/RConn1 -- Current Measurement3/RConn1 -- Voltage Measurement1/LConn2 -- 1-/RConn1
  2+/RConn1 -- Current Measurement3/LConn1 -- Voltage Measurement2/LConn1
  Voltage Measurement2/LConn2 -- Current Measurement4/RConn1 -- 1_out/RConn1 -- 2-/RConn1

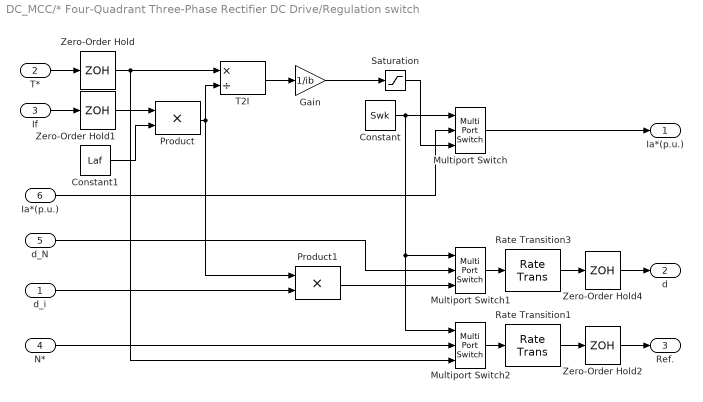
== system DC_MCC/* Four-Quadrant Three-Phase Rectifier DC Drive/Regulation switch ==
  d_i : Inport
  T* : Inport  Port=2
  If : Inport  Port=3
  N* : Inport  Port=4
  d_N : Inport  Port=5
  Ia*(p.u.) : Inport  Port=6
  Constant : Constant  Value=Swk
  Constant1 : Constant  Value=Laf
  Gain : Gain  Gain=1/ib  SaturateOnIntegerOverflow=on  OutDataTypeStr=Inherit: Same as input  ParamDataTypeStr=Inherit: Same as input
  Multiport Switch : MultiPortSwitch  Inputs=2  SaturateOnIntegerOverflow=on
  Multiport Switch1 : MultiPortSwitch  Inputs=2  SaturateOnIntegerOverflow=on
  Multiport Switch2 : MultiPortSwitch  Inputs=2  SaturateOnIntegerOverflow=on
  Product : Product  SaturateOnIntegerOverflow=on  OutDataTypeStr=Inherit: Same as first input
  Product1 : Product  SaturateOnIntegerOverflow=on  OutDataTypeStr=Inherit: Same as first input
  Rate Transition1 : RateTransition
  Rate Transition3 : RateTransition
  Saturation : Saturate  UpperLimit=lim  LowerLimit=-lim
  T2I : Product  Inputs=*/  SaturateOnIntegerOverflow=on  OutDataTypeStr=Inherit: Same as first input
  Zero-Order Hold : ZeroOrderHold  SampleTime=sampling
  Zero-Order Hold1 : ZeroOrderHold  SampleTime=sampling
  Zero-Order Hold2 : ZeroOrderHold  SampleTime=Ts
  Zero-Order Hold4 : ZeroOrderHold  SampleTime=Ts
  " Ia*(p.u.)" : Outport
  d : Outport  Port=2
  Ref. : Outport  Port=3
  wires:
  Product1/1 -> Multiport Switch1/3
  d_N/1 -> Multiport Switch1/2
  T2I/1 -> Gain/1
  Saturation/1 -> Multiport Switch/3
  Gain/1 -> Saturation/1
  Zero-Order Hold/1 -> Multiport Switch2/3, T2I/1
  T*/1 -> Zero-Order Hold/1
  If/1 -> Zero-Order Hold1/1
  Constant/1 -> Multiport Switch2/1, Multiport Switch1/1, Multiport Switch/1
  Zero-Order Hold1/1 -> Product/1
  Product/1 -> T2I/2, Product1/1
  Constant1/1 -> Product/2
  Rate Transition3/1 -> Zero-Order Hold4/1
  Zero-Order Hold4/1 -> d/1
  Multiport Switch1/1 -> Rate Transition3/1
  d_i/1 -> Product1/2
  Rate Transition1/1 -> Zero-Order Hold2/1
  Zero-Order Hold2/1 -> Ref./1
  Multiport Switch2/1 -> Rate Transition1/1
  N*/1 -> Multiport Switch2/2
  Multiport Switch/1 -> " Ia*(p.u.)"/1
  Ia*(p.u.)/1 -> Multiport Switch/2

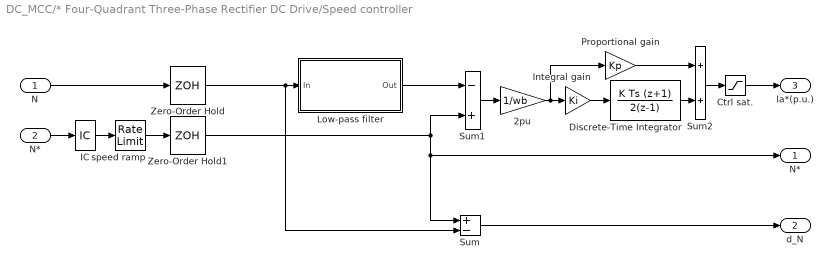
== system DC_MCC/* Four-Quadrant Three-Phase Rectifier DC Drive/Speed controller ==
  N : Inport
  N* : Inport  Port=2
  2pu : Gain  Gain=1/wb  SaturateOnIntegerOverflow=on  OutDataTypeStr=Inherit: Same as input  ParamDataTypeStr=Inherit: Same as input
  Ctrl sat. : Saturate  UpperLimit=lim  LowerLimit=-lim
  Discrete-Time Integrator : DiscreteIntegrator  IntegratorMethod=Integration: Trapezoidal  SampleTime=sampling  LimitOutput=on  UpperSaturationLimit=lim  LowerSaturationLimit=-lim  ICPrevOutput=DiscIntNeverNeededParam  ICPrevScaledInput=DiscIntNeverNeededParam
  IC : InitialCondition  Value=Is
  Integral gain : Gain  Gain=Ki  SaturateOnIntegerOverflow=on  OutDataTypeStr=Inherit: Same as input  ParamDataTypeStr=Inherit: Same as input
  Low-pass filter : Subsystem
  Proportional gain : Gain  Gain=Kp  SaturateOnIntegerOverflow=on  OutDataTypeStr=Inherit: Same as input  ParamDataTypeStr=Inherit: Same as input
  Sum : Sum  Inputs=+-  SaturateOnIntegerOverflow=on  InputSameDT=on  OutDataTypeStr=Inherit: Same as first input
  Sum1 : Sum  Inputs=-+  SaturateOnIntegerOverflow=on  InputSameDT=on  OutDataTypeStr=Inherit: Same as first input
  Sum2 : Sum  SaturateOnIntegerOverflow=on  InputSameDT=on  OutDataTypeStr=Inherit: Same as first input
  Zero-Order Hold : ZeroOrderHold  SampleTime=sampling
  Zero-Order Hold1 : ZeroOrderHold  SampleTime=sampling
  speed ramp : RateLimiter  RisingSlewLimit=ramp(2)  FallingSlewLimit=ramp(1)
  " N*" : Outport  InitialOutput=0
  d_N : Outport  Port=2  InitialOutput=0
  Ia*(p.u.) : Outport  Port=3  InitialOutput=0
  wires:
  speed ramp/1 -> Zero-Order Hold1/1
  Ctrl sat./1 -> Ia*(p.u.)/1
  2pu/1 -> Integral gain/1, Proportional gain/1
  Sum1/1 -> 2pu/1
  Proportional gain/1 -> Sum2/1
  Integral gain/1 -> Discrete-Time Integrator/1
  Discrete-Time Integrator/1 -> Sum2/2
  Sum2/1 -> Ctrl sat./1
  Sum/1 -> d_N/1
  Low-pass filter/1(Out) -> Sum1/1
  N*/1 -> IC/1
  IC/1 -> speed ramp/1
  N/1 -> Zero-Order Hold/1
  Zero-Order Hold/1 -> Sum/2, Low-pass filter/1(In)
  Zero-Order Hold1/1 -> " N*"/1, Sum/1, Sum1/2

== system DC_MCC/* Four-Quadrant Three-Phase Rectifier DC Drive/Subsystem ==
  Va : Inport
  m : Inport  Port=2
  1\ib1 : Gain  Gain=30/pi  SaturateOnIntegerOverflow=on  OutDataTypeStr=Inherit: Same as input  ParamDataTypeStr=Inherit: Same as input
  Bus Creator3 : BusCreator  Inputs=5
  Bus Selector : BusSelector  OutputSignals=Speed wm (rad/s),Armature current ia (A),Field current if (A),Electrical torque Te (n m)
  Motor : Outport
  wires:
  Bus Selector/1 -> 1\ib1/1  "<Speed wm (rad/s)>"
  m/1 -> Bus Selector/1
  Va/1 -> Bus Creator3/1  "Armature Voltage (V)"
  Bus Creator3/1 -> Motor/1
  Bus Selector/2 -> Bus Creator3/3  "<Armature current ia (A)>"
  Bus Selector/3 -> Bus Creator3/4  "<Field current if (A)>"
  1\ib1/1 -> Bus Creator3/2  "Speed (rpm)"
  Bus Selector/4 -> Bus Creator3/5  "<Electrical torque Te (n m)>"

== system DC_MCC/* Four-Quadrant Three-Phase Rectifier DC Drive/Bridge driver/Crossover timer_1 ==
  In1 : Inport
  Constant3 : Constant  Value=time
  Digital Clock : DigitalClock  SampleTime=sampling
  Logical Operator15 : Logic  Operator=NOT
  Relational Operator4 : RelationalOperator  Operator=>  RndMeth=Nearest  InputSameDT=on
  Sum2 : Sum  Inputs=+-  SaturateOnIntegerOverflow=on  InputSameDT=on  OutDataTypeStr=Inherit: Same as first input
  Switch3 : Switch  Threshold=0.5  SaturateOnIntegerOverflow=on  InputSameDT=on
  Unit Delay2 : UnitDelay  SampleTime=sampling
  Out1 : Outport
  wires:
  Logical Operator15/1 -> Switch3/2
  In1/1 -> Logical Operator15/1
  Relational Operator4/1 -> Out1/1
  Constant3/1 -> Relational Operator4/2
  Sum2/1 -> Relational Operator4/1
  Unit Delay2/1 -> Switch3/3
  Digital Clock/1 -> Sum2/1, Switch3/1
  Switch3/1 -> Sum2/2, Unit Delay2/1

== system DC_MCC/* Four-Quadrant Three-Phase Rectifier DC Drive/Bridge driver/Crossover timer_2 ==
  In1 : Inport
  Constant3 : Constant  Value=time
  Digital Clock : DigitalClock  SampleTime=sampling
  Logical Operator15 : Logic  Operator=NOT
  Relational Operator4 : RelationalOperator  Operator=>  RndMeth=Nearest  InputSameDT=on
  Sum2 : Sum  Inputs=+-  SaturateOnIntegerOverflow=on  InputSameDT=on  OutDataTypeStr=Inherit: Same as first input
  Switch3 : Switch  Threshold=0.5  SaturateOnIntegerOverflow=on  InputSameDT=on
  Unit Delay2 : UnitDelay  SampleTime=sampling
  Out1 : Outport
  wires:
  Switch3/1 -> Unit Delay2/1, Sum2/2
  Digital Clock/1 -> Switch3/1, Sum2/1
  Unit Delay2/1 -> Switch3/3
  Sum2/1 -> Relational Operator4/1
  Constant3/1 -> Relational Operator4/2
  Relational Operator4/1 -> Out1/1
  In1/1 -> Logical Operator15/1
  Logical Operator15/1 -> Switch3/2

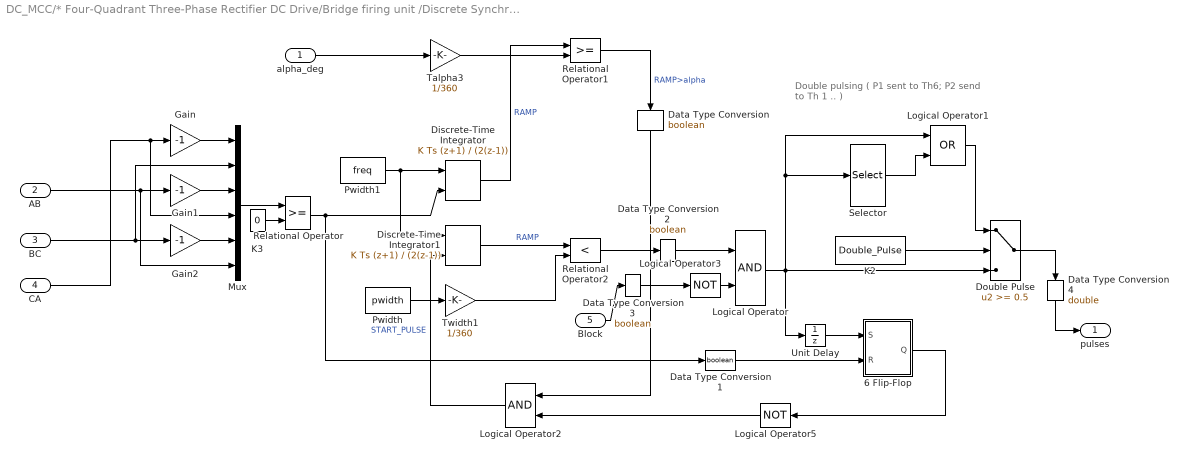
== system DC_MCC/* Four-Quadrant Three-Phase Rectifier DC Drive/Bridge firing unit /Discrete Synchronized 6-Pulse Generator2 ==
  note: Double pulsing
      |  ( P1 sent to  Th6;  P2 send to Th 1 .. )
  alpha_deg : Inport
  AB : Inport  Port=2
  BC : Inport  Port=3
  CA : Inport  Port=4
  Block : Inport  Port=5
  6 Flip-Flop : Subsystem
  Data Type Conversion{,1..3} (4 alike) : DataTypeConversion  OutDataTypeStr=boolean  SaturateOnIntegerOverflow=on  RndMeth=Zero
  Data Type Conversion4 : DataTypeConversion  OutDataTypeStr=double  SaturateOnIntegerOverflow=on  RndMeth=Zero
  Discrete-Time Integrator : DiscreteIntegrator  IntegratorMethod=Integration: Trapezoidal  ExternalReset=rising  SampleTime=Ts  ICPrevOutput=DiscIntNeverNeededParam  ICPrevScaledInput=DiscIntNeverNeededParam
  Discrete-Time Integrator1 : DiscreteIntegrator  IntegratorMethod=Integration: Trapezoidal  ExternalReset=rising  SampleTime=Ts  ICPrevOutput=DiscIntNeverNeededParam  ICPrevScaledInput=DiscIntNeverNeededParam
  Double Pulse : Switch  Threshold=0.5  SaturateOnIntegerOverflow=on  InputSameDT=on
  Gain : Gain  Gain=-1  SaturateOnIntegerOverflow=on  OutDataTypeStr=Inherit: Same as input  ParamDataTypeStr=Inherit: Same as input
  Gain1 : Gain  Gain=-1  SaturateOnIntegerOverflow=on  OutDataTypeStr=Inherit: Same as input  ParamDataTypeStr=Inherit: Same as input
  Gain2 : Gain  Gain=-1  SaturateOnIntegerOverflow=on  OutDataTypeStr=Inherit: Same as input  ParamDataTypeStr=Inherit: Same as input
  K2 : Constant  Value=Double_Pulse
  K3 : Constant  Value=0
  Logical Operator : Logic
  Logical Operator1 : Logic  Operator=OR
  Logical Operator2 : Logic
  Logical Operator3 : Logic  Operator=NOT  Inputs=1
  Logical Operator5 : Logic  Operator=NOT  Inputs=1
  Mux : Mux  Inputs=6
  Pwidth : Constant  Value=pwidth
  Pwidth1 : Constant  Value=freq
  Relational Operator : RelationalOperator  RndMeth=Nearest  InputSameDT=on
  Relational Operator1 : RelationalOperator  RndMeth=Nearest  InputSameDT=on
  Relational Operator2 : RelationalOperator  Operator=<  RndMeth=Nearest  InputSameDT=on
  Selector : Selector  InputPortWidth=6  IndexOptions=Index vector (dialog)  Indices=[2 3 4 5 6 1 ]  OutputSizes=1
  Talpha3 : Gain  Gain=1/360  SaturateOnIntegerOverflow=on  OutDataTypeStr=Inherit: Same as input  ParamDataTypeStr=Inherit: Same as input
  Twidth1 : Gain  Gain=1/360  SaturateOnIntegerOverflow=on  OutDataTypeStr=Inherit: Same as input  ParamDataTypeStr=Inherit: Same as input
  Unit Delay : UnitDelay  SampleTime=Ts
  pulses : Outport  InitialOutput=0
  wires:
  Data Type Conversion4/1 -> pulses/1
  Double Pulse/1 -> Data Type Conversion4/1
  Data Type Conversion3/1 -> Logical Operator3/1
  Block/1 -> Data Type Conversion3/1
  Data Type Conversion2/1 -> Logical Operator/1
  Relational Operator2/1 -> Data Type Conversion2/1
  Data Type Conversion1/1 -> 6 Flip-Flop/2(R)
  Data Type Conversion/1 -> Logical Operator2/1
  Relational Operator1/1 -> Data Type Conversion/1  "RAMP>alpha"
  Logical Operator2/1 -> Discrete-Time Integrator1/2  "START_PULSE"
  AB/1 -> Mux/6, Gain1/1
  Logical Operator3/1 -> Logical Operator/2
  Unit Delay/1 -> 6 Flip-Flop/1(S)
  K2/1 -> Double Pulse/2
  Logical Operator/1 -> Unit Delay/1, Double Pulse/3, Selector/1, Logical Operator1/1
  Selector/1 -> Logical Operator1/2
  Logical Operator1/1 -> Double Pulse/1
  Pwidth/1 -> Twidth1/1
  Twidth1/1 -> Relational Operator2/2
  Discrete-Time Integrator1/1 -> Relational Operator2/1  "RAMP"
  Discrete-Time Integrator/1 -> Relational Operator1/1  "RAMP"
  Gain/1 -> Mux/1
  Gain1/1 -> Mux/3
  Gain2/1 -> Mux/5
  K3/1 -> Relational Operator/2
  Relational Operator/1 -> Data Type Conversion1/1, Discrete-Time Integrator/2
  Logical Operator5/1 -> Logical Operator2/2
  Talpha3/1 -> Relational Operator1/2
  Mux/1 -> Relational Operator/1
  CA/1 -> Gain/1, Mux/4
  BC/1 -> Gain2/1, Mux/2
  Pwidth1/1 -> Discrete-Time Integrator/1, Discrete-Time Integrator1/1
  6 Flip-Flop/1(Q) -> Logical Operator5/1
  alpha_deg/1 -> Talpha3/1

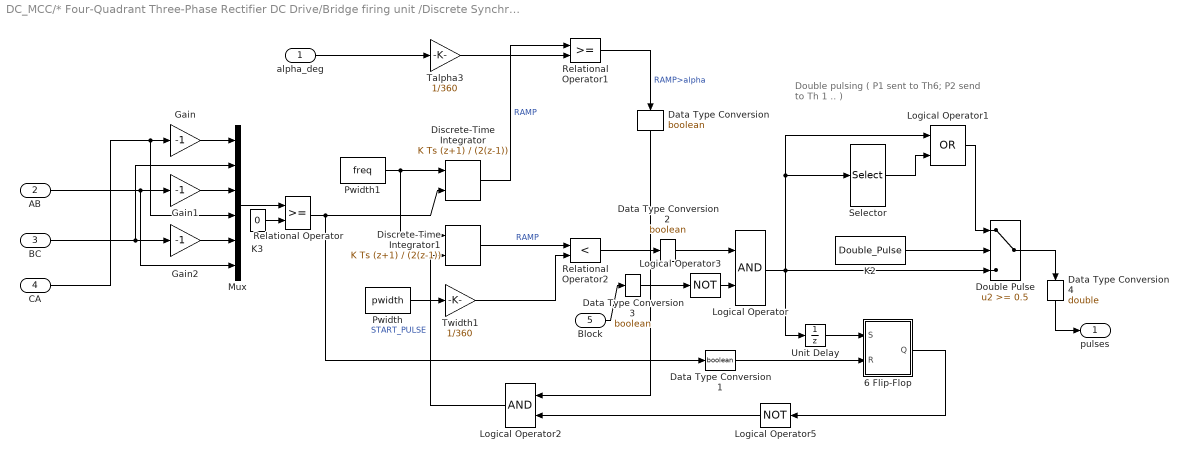
== system DC_MCC/* Four-Quadrant Three-Phase Rectifier DC Drive/Bridge firing unit /Discrete Synchronized 6-Pulse Generator3 ==
  note: Double pulsing
      |  ( P1 sent to  Th6;  P2 send to Th 1 .. )
  alpha_deg : Inport
  AB : Inport  Port=2
  BC : Inport  Port=3
  CA : Inport  Port=4
  Block : Inport  Port=5
  6 Flip-Flop : Subsystem
  Data Type Conversion{,1..3} (4 alike) : DataTypeConversion  OutDataTypeStr=boolean  SaturateOnIntegerOverflow=on  RndMeth=Zero
  Data Type Conversion4 : DataTypeConversion  OutDataTypeStr=double  SaturateOnIntegerOverflow=on  RndMeth=Zero
  Discrete-Time Integrator : DiscreteIntegrator  IntegratorMethod=Integration: Trapezoidal  ExternalReset=rising  SampleTime=Ts  ICPrevOutput=DiscIntNeverNeededParam  ICPrevScaledInput=DiscIntNeverNeededParam
  Discrete-Time Integrator1 : DiscreteIntegrator  IntegratorMethod=Integration: Trapezoidal  ExternalReset=rising  SampleTime=Ts  ICPrevOutput=DiscIntNeverNeededParam  ICPrevScaledInput=DiscIntNeverNeededParam
  Double Pulse : Switch  Threshold=0.5  SaturateOnIntegerOverflow=on  InputSameDT=on
  Gain : Gain  Gain=-1  SaturateOnIntegerOverflow=on  OutDataTypeStr=Inherit: Same as input  ParamDataTypeStr=Inherit: Same as input
  Gain1 : Gain  Gain=-1  SaturateOnIntegerOverflow=on  OutDataTypeStr=Inherit: Same as input  ParamDataTypeStr=Inherit: Same as input
  Gain2 : Gain  Gain=-1  SaturateOnIntegerOverflow=on  OutDataTypeStr=Inherit: Same as input  ParamDataTypeStr=Inherit: Same as input
  K2 : Constant  Value=Double_Pulse
  K3 : Constant  Value=0
  Logical Operator : Logic
  Logical Operator1 : Logic  Operator=OR
  Logical Operator2 : Logic
  Logical Operator3 : Logic  Operator=NOT  Inputs=1
  Logical Operator5 : Logic  Operator=NOT  Inputs=1
  Mux : Mux  Inputs=6
  Pwidth : Constant  Value=pwidth
  Pwidth1 : Constant  Value=freq
  Relational Operator : RelationalOperator  RndMeth=Nearest  InputSameDT=on
  Relational Operator1 : RelationalOperator  RndMeth=Nearest  InputSameDT=on
  Relational Operator2 : RelationalOperator  Operator=<  RndMeth=Nearest  InputSameDT=on
  Selector : Selector  InputPortWidth=6  IndexOptions=Index vector (dialog)  Indices=[2 3 4 5 6 1 ]  OutputSizes=1
  Talpha3 : Gain  Gain=1/360  SaturateOnIntegerOverflow=on  OutDataTypeStr=Inherit: Same as input  ParamDataTypeStr=Inherit: Same as input
  Twidth1 : Gain  Gain=1/360  SaturateOnIntegerOverflow=on  OutDataTypeStr=Inherit: Same as input  ParamDataTypeStr=Inherit: Same as input
  Unit Delay : UnitDelay  SampleTime=Ts
  pulses : Outport  InitialOutput=0
  wires:
  alpha_deg/1 -> Talpha3/1
  6 Flip-Flop/1(Q) -> Logical Operator5/1
  Pwidth1/1 -> Discrete-Time Integrator1/1, Discrete-Time Integrator/1
  BC/1 -> Mux/2, Gain2/1
  CA/1 -> Mux/4, Gain/1
  Mux/1 -> Relational Operator/1
  Talpha3/1 -> Relational Operator1/2
  Logical Operator5/1 -> Logical Operator2/2
  Relational Operator/1 -> Discrete-Time Integrator/2, Data Type Conversion1/1
  K3/1 -> Relational Operator/2
  Gain2/1 -> Mux/5
  Gain1/1 -> Mux/3
  Gain/1 -> Mux/1
  Discrete-Time Integrator/1 -> Relational Operator1/1  "RAMP"
  Discrete-Time Integrator1/1 -> Relational Operator2/1  "RAMP"
  Twidth1/1 -> Relational Operator2/2
  Pwidth/1 -> Twidth1/1
  Logical Operator1/1 -> Double Pulse/1
  Selector/1 -> Logical Operator1/2
  Logical Operator/1 -> Logical Operator1/1, Selector/1, Double Pulse/3, Unit Delay/1
  K2/1 -> Double Pulse/2
  Unit Delay/1 -> 6 Flip-Flop/1(S)
  Logical Operator3/1 -> Logical Operator/2
  AB/1 -> Gain1/1, Mux/6
  Logical Operator2/1 -> Discrete-Time Integrator1/2  "START_PULSE"
  Relational Operator1/1 -> Data Type Conversion/1  "RAMP>alpha"
  Data Type Conversion/1 -> Logical Operator2/1
  Data Type Conversion1/1 -> 6 Flip-Flop/2(R)
  Relational Operator2/1 -> Data Type Conversion2/1
  Data Type Conversion2/1 -> Logical Operator/1
  Block/1 -> Data Type Conversion3/1
  Data Type Conversion3/1 -> Logical Operator3/1
  Double Pulse/1 -> Data Type Conversion4/1
  Data Type Conversion4/1 -> pulses/1
